simulink model "DFL_IMAP"  (R2018b)
(part 4 of 5)

  Gain384/1 -> Data Type Conversion560/1, IMAPve_g_ORI_L1_ExistProb/1  "IMAPve_g_ORI_L1_ExistProb"
  message_unpack/125(IFC_Line03_LineID) -> Gain383/1
  message_unpack/127(IFC_Line03_DxStart) -> Gain381/1
  Gain381/1 -> Data Type Conversion561/1, IMAPve_g_ORI_L1_Dxstart/1  "IMAPve_g_ORI_L1_Dxstart"
  message_unpack/124(IFC_Line02_TypeConf) -> Gain380/1
  Data Type Conversion560/1 -> Terminator453/1  "ob_IMAPve_g_ORI_L1_ExistProb"
  Data Type Conversion562/1 -> Terminator455/1  "ob_IMAPve_d_ORI_L1_ColorClass"
  Data Type Conversion559/1 -> Terminator452/1  "ob_IMAPve_d_ORI_L1_ID"
  Gain382/1 -> Data Type Conversion562/1, IMAPve_d_ORI_L1_ColorClass/1  "IMAPve_d_ORI_L1_ColorClass"
  message_unpack/128(IFC_Line03_ColorClass) -> Gain382/1
  Data Type Conversion561/1 -> Terminator454/1  "ob_IMAPve_g_ORI_L1_Dxstart"
  Gain383/1 -> Data Type Conversion559/1, IMAPve_d_ORI_L1_ID/1  "IMAPve_d_ORI_L1_ID"
  Data Type Conversion557/1 -> Terminator451/1  "ob_IMAPve_g_ORI_R0_TypeConf"
  Gain379/1 -> Data Type Conversion563/1, IMAPve_d_ORI_L1_MeasureType/1  "IMAPve_d_ORI_L1_MeasureType"
  message_unpack/134(IFC_Line03_MeasureType) -> Gain379/1
  Data Type Conversion563/1 -> Terminator456/1  "ob_IMAPve_d_ORI_L1_MeasureType"
  Gain377/1 -> Data Type Conversion564/1, IMAPve_g_ORI_L1_TypeConf/1  "IMAPve_g_ORI_L1_TypeConf"
  Gain375/1 -> Data Type Conversion567/1, IMAPve_g_ORI_R1_Dxstart/1  "IMAPve_g_ORI_R1_Dxstart"
  message_unpack/138(IFC_Line04_LineID) -> Gain378/1
  Gain376/1 -> Data Type Conversion566/1, IMAPve_g_ORI_R1_ExistProb/1  "IMAPve_g_ORI_R1_ExistProb"
  Gain374/1 -> Data Type Conversion568/1, IMAPve_d_ORI_R1_ColorClass/1  "IMAPve_d_ORI_R1_ColorClass"
  message_unpack/137(IFC_Line03_TypeConf) -> Gain377/1
  Data Type Conversion567/1 -> Terminator465/1  "ob_IMAPve_g_ORI_R1_Dxstart"
  Gain378/1 -> Data Type Conversion565/1, IMAPve_d_ORI_R1_ID/1  "IMAPve_d_ORI_R1_ID"
  message_unpack/140(IFC_Line04_DxStart) -> Gain375/1
  Data Type Conversion568/1 -> Terminator466/1  "ob_IMAPve_d_ORI_R1_ColorClass"
  message_unpack/139(IFC_Line04_ExistProb) -> Gain376/1
  Data Type Conversion564/1 -> Terminator462/1  "ob_IMAPve_g_ORI_L1_TypeConf"
  Data Type Conversion565/1 -> Terminator463/1  "ob_IMAPve_d_ORI_R1_ID"
  message_unpack/141(IFC_Line04_ColorClass) -> Gain374/1
  Data Type Conversion566/1 -> Terminator464/1  "ob_IMAPve_g_ORI_R1_ExistProb"
  message_unpack/147(IFC_Line04_MeasureType) -> Gain373/1
  Gain373/1 -> Data Type Conversion569/1, IMAPve_d_ORI_R1_MeasureType/1  "IMAPve_d_ORI_R1_MeasureType"
  Data Type Conversion569/1 -> Terminator457/1  "ob_IMAPve_d_ORI_R1_MeasureType"
  message_unpack/150(IFC_Line04_TypeConf) -> Gain/1
  Gain/1 -> Data Type Conversion590/1, IMAPve_g_ORI_R1_TypeConf/1  "IMAPve_g_ORI_R1_TypeConf"
  Data Type Conversion590/1 -> Terminator483/1  "ob_IMAPve_g_ORI_R1_TypeConf"
  message_unpack/162(IFC_Roadedge02_ExistProb) -> Gain364/1
  Gain361/1 -> Data Type Conversion579/1, IMAPve_d_ORI_RoadedgeL0_MeasureType/1  "IMAPve_d_ORI_RoadedgeL0_MeasureType"
  Gain357/1 -> Data Type Conversion576/1, IMAPve_g_ORI_RoadedgeL0_C0/1  "IMAPve_g_ORI_RoadedgeL0_C0"
  message_unpack/163(IFC_Roadedge02_DxStart) -> Gain365/1
  Gain354/1 -> Data Type Conversion573/1, IMAPve_g_ORI_RoadedgeL0_DxStart/1  "IMAPve_g_ORI_RoadedgeL0_DxStart"
  Gain369/1 -> Data Type Conversion586/1, IMAPve_g_ORI_RoadedgeR0_C3/1  "IMAPve_g_ORI_RoadedgeR0_C3"
  Gain365/1 -> Data Type Conversion578/1, IMAPve_g_ORI_RoadedgeR0_DxStart/1  "IMAPve_g_ORI_RoadedgeR0_DxStart"
  Gain360/1 -> Data Type Conversion571/1, IMAPve_g_ORI_RoadedgeL0_C2/1  "IMAPve_g_ORI_RoadedgeL0_C2"
  message_unpack/168(IFC_Roadedge02_CurvChange) -> Gain370/1
  message_unpack/155(IFC_Roadedge01_HeadingAngle) -> Gain356/1
  Gain363/1 -> IMAPve_d_ORI_RoadedgeR0_ID/1, Data Type Conversion581/1  "IMAPve_d_ORI_RoadedgeR0_ID"
  message_unpack/158(IFC_Roadedge01_CurvChange) -> Gain360/1
  message_unpack/152(IFC_Roadedge01_ExistProb) -> Gain288/1
  Gain366/1 -> Data Type Conversion583/1, IMAPve_g_ORI_RoadedgeR0_DxEnd/1  "IMAPve_g_ORI_RoadedgeR0_DxEnd"
  Gain356/1 -> Data Type Conversion575/1, IMAPve_g_ORI_RoadedgeL0_C1/1  "IMAPve_g_ORI_RoadedgeL0_C1"
  Gain371/1 -> Data Type Conversion588/1, IMAPve_d_ORI_RoadedgeR0_MeasureType/1  "IMAPve_d_ORI_RoadedgeR0_MeasureType"
  message_unpack/169(IFC_Roadedge02_MeasureType) -> Gain371/1
  Gain367/1 -> Data Type Conversion584/1, IMAPve_g_ORI_RoadedgeR0_C1/1  "IMAPve_g_ORI_RoadedgeR0_C1"
  Gain364/1 -> Data Type Conversion582/1, IMAPve_g_ORI_RoadedgeR0_ExistProb/1  "IMAPve_g_ORI_RoadedgeR0_ExistProb"
  message_unpack/170(IFC_Roadedge02_Type) -> Gain372/1
  message_unpack/159(IFC_Roadedge01_MeasureType) -> Gain361/1
  message_unpack/160(IFC_Roadedge01_Type) -> Gain362/1
  message_unpack/157(IFC_Roadedge01_Curv) -> Gain359/1
  Gain355/1 -> Data Type Conversion574/1, IMAPve_g_ORI_RoadedgeL0_DxEnd/1  "IMAPve_g_ORI_RoadedgeL0_DxEnd"
  message_unpack/156(IFC_Roadedge01_Dy) -> Gain357/1
  Data Type Conversion584/1 -> Terminator477/1  "ob_IMAPve_g_ORI_RoadedgeR0_C1"
  Data Type Conversion589/1 -> Terminator482/1  "ob_IMAPve_d_ORI_RoadedgeR0_Type"
  Data Type Conversion580/1 -> Terminator473/1  "ob_IMAPve_d_ORI_RoadedgeL0_Type"
  Data Type Conversion585/1 -> Terminator478/1  "ob_IMAPve_g_ORI_RoadedgeR0_C0"
  Data Type Conversion588/1 -> Terminator481/1  "ob_IMAPve_d_ORI_RoadedgeR0_MeasureType"
  Gain372/1 -> Data Type Conversion589/1, IMAPve_d_ORI_RoadedgeR0_Type/1  "IMAPve_d_ORI_RoadedgeR0_Type"
  Data Type Conversion574/1 -> Terminator467/1  "ob_IMAPve_g_ORI_RoadedgeL0_DxEnd"
  Data Type Conversion582/1 -> Terminator475/1  "ob_IMAPve_g_ORI_RoadedgeR0_ExistProb"
  Data Type Conversion576/1 -> Terminator469/1  "ob_IMAPve_g_ORI_RoadedgeL0_C0"
  Data Type Conversion581/1 -> Terminator474/1  "ob_IMAPve_d_ORI_RoadedgeR0_ID"
  Data Type Conversion570/1 -> Terminator458/1  "ob_IMAPve_d_ORI_RoadedgeL0_ID"
  message_unpack/153(IFC_Roadedge01_DxStart) -> Gain354/1
  message_unpack/166(IFC_Roadedge02_Dy) -> Gain368/1
  Data Type Conversion577/1 -> Terminator470/1  "ob_IMAPve_g_ORI_RoadedgeL0_C3"
  Data Type Conversion586/1 -> Terminator479/1  "ob_IMAPve_g_ORI_RoadedgeR0_C3"
  Data Type Conversion578/1 -> Terminator471/1  "ob_IMAPve_g_ORI_RoadedgeR0_DxStart"
  Data Type Conversion583/1 -> Terminator476/1  "ob_IMAPve_g_ORI_RoadedgeR0_DxEnd"
  Data Type Conversion572/1 -> Terminator460/1  "ob_IMAPve_g_ORI_RoadedgeL0_ExistProb"
  Data Type Conversion575/1 -> Terminator468/1  "ob_IMAPve_g_ORI_RoadedgeL0_C1"
  Data Type Conversion579/1 -> Terminator472/1  "ob_IMAPve_d_ORI_RoadedgeL0_MeasureType"
  Data Type Conversion571/1 -> Terminator459/1  "ob_IMAPve_g_ORI_RoadedgeL0_C2"
  message_unpack/154(IFC_Roadedge01_DxEnd) -> Gain355/1
  message_unpack/164(IFC_Roadedge02_DxEnd) -> Gain366/1
  message_unpack/165(IFC_Roadedge02_HeadingAngle) -> Gain367/1
  message_unpack/151(IFC_Roadedge01_LineID) -> Gain358/1
  message_unpack/161(IFC_Roadedge02_LineID) -> Gain363/1
  Gain370/1 -> Data Type Conversion587/1, IMAPve_g_ORI_RoadedgeR0_C2/1  "IMAPve_g_ORI_RoadedgeR0_C2"
  message_unpack/167(IFC_Roadedge02_Curv) -> Gain369/1
  Gain358/1 -> Data Type Conversion570/1, IMAPve_d_ORI_RoadedgeL0_ID/1  "IMAPve_d_ORI_RoadedgeL0_ID"
  Data Type Conversion573/1 -> Terminator461/1  "ob_IMAPve_g_ORI_RoadedgeL0_DxStart"
  Gain288/1 -> Data Type Conversion572/1, IMAPve_g_ORI_RoadedgeL0_ExistProb/1  "IMAPve_g_ORI_RoadedgeL0_ExistProb"
  Data Type Conversion587/1 -> Terminator480/1  "ob_IMAPve_g_ORI_RoadedgeR0_C2"
  Gain359/1 -> Data Type Conversion577/1, IMAPve_g_ORI_RoadedgeL0_C3/1  "IMAPve_g_ORI_RoadedgeL0_C3"
  Gain362/1 -> Data Type Conversion580/1, IMAPve_d_ORI_RoadedgeL0_Type/1  "IMAPve_d_ORI_RoadedgeL0_Type"
  Gain368/1 -> Data Type Conversion585/1, IMAPve_g_ORI_RoadedgeR0_C0/1  "IMAPve_g_ORI_RoadedgeR0_C0"
  CAFDva_y_F_CameraData47E/1 -> message_unpack/50(CAFDva_y_F_CameraData47E)
  array_transfer/1(output) -> Gain3/1
  array_transfer8/1(output) -> Gain5/1
  array_transfer3/1(output) -> Gain8/1
  Data Type Conversion48/1 -> Terminator39/1  "ob_IMAPve_d_SCC_Left_SwitchSig"
